simulink model "PID_Model"  (Simulink 8.7)
settings: Solver=ode15s  StartTime=0.0  StopTime=20  RelTol=1e-6
undefined symbols (not defined in the file or in its folder): Kd, Ki, Kp
settings Model: Creator=tongji_HEV  LastModifiedBy=Mor
settings DataIOCC: SignalLoggingSaveFormat=ModelDataLogs  SignalLoggingName=sigsOut
settings OptimizationCC: ExpressionDepthLimit=2147483647  InitFltsAndDblsToZero=on
settings DebuggingCC: SaveWithParameterizedLinksMsg=none  SignalResolutionControl=TryResolveAllWithWarning  MultiTaskDSMMsg=warning  MultiTaskCondExecSysMsg=none  FcnCallInpInsideContextMsg=UseLocalSettings  StateNameClashWarn=warning  StrictBusMsg=None
settings HardwareCC: TargetUnknown=on
settings GRTTargetCC: TargetFcnLib=ansi_tfl_tmw.mat  GeneratePreprocessorConditionals=Use local settings  CombineOutputUpdateFcns=off  GRTInterface=on

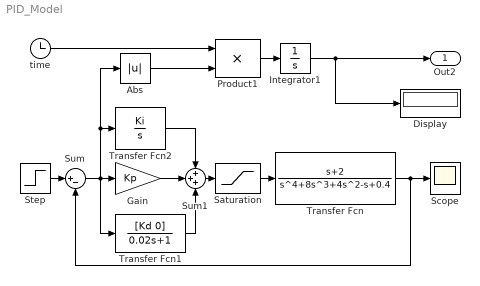
== system PID_Model ==
  Abs : Abs  ZeroCross=off  SaturateOnIntegerOverflow=on
  Display : Display
  Gain : Gain  Gain=Kp
  Integrator1 : Integrator
  Product1 : Product  SaturateOnIntegerOverflow=on  OutDataTypeStr=Inherit: Same as first input
  Saturation : Saturate  UpperLimit=5  LowerLimit=-5
  Scope : Scope
  Step : Step  Time=0  SampleTime=0
  Sum : Sum  Inputs=|+-  SaturateOnIntegerOverflow=on
  Sum1 : Sum  Inputs=+++  SaturateOnIntegerOverflow=on
  Transfer Fcn : TransferFcn  Numerator=[1 2 ]  Denominator=[1 8 4 -1 0.4]
  Transfer Fcn1 : TransferFcn  Numerator=[Kd 0]  Denominator=[0.02 1 ]
  Transfer Fcn2 : TransferFcn  Numerator=Ki  Denominator=[1 0 ]
  time : Clock
  Out2 : Outport
  wires:
  Step/1 -> Sum/1
  Sum/1 -> Transfer Fcn1/1, Gain/1, Abs/1, Transfer Fcn2/1
  Transfer Fcn/1 -> Scope/1, Sum/2
  time/1 -> Product1/1
  Integrator1/1 -> Out2/1, Display/1
  Product1/1 -> Integrator1/1
  Abs/1 -> Product1/2
  Sum1/1 -> Saturation/1
  Saturation/1 -> Transfer Fcn/1
  Gain/1 -> Sum1/2
  Transfer Fcn1/1 -> Sum1/3
  Transfer Fcn2/1 -> Sum1/1
